simulink model "lab03fig2a"  (R2015a)
settings: Solver=ode45  StartTime=0.0  StopTime=20.0  RelTol=1e-3
settings Model: Creator=dg  LastModifiedBy=dg

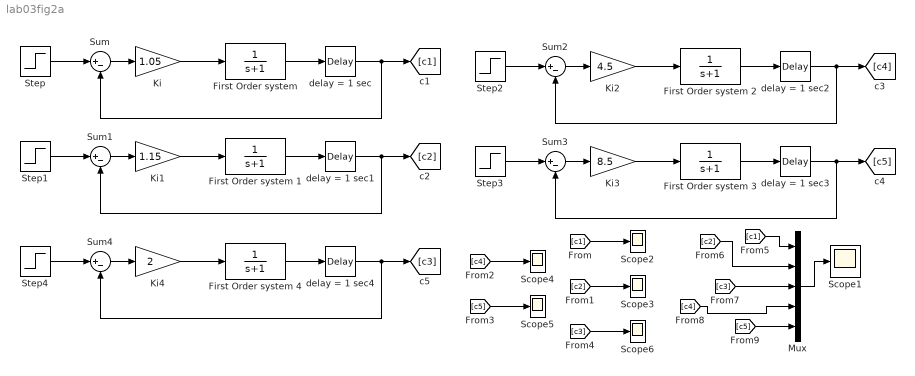
== system lab03fig2a ==
  First Order system {,1..4} (5 alike) : TransferFcn  Denominator=[1 1]
  Ki : Gain  Gain=1.05
  Ki1 : Gain  Gain=1.15
  Ki2 : Gain  Gain=4.5
  Ki3 : Gain  Gain=8.5
  Ki4 : Gain  Gain=2
  Mux : Mux  Inputs=5
  Scope{1..6} (6 alike) : Scope
      Scope1 settings: TickLabels=on  YMin=-1  YMax=4
      Scope2 settings: TickLabels=on  YMin=-1  YMax=4
      Scope3 settings: TickLabels=on  YMin=-1  YMax=4  SaveName=ScopeData2
      Scope4 settings: TickLabels=on  YMin=-1  YMax=4  SaveName=ScopeData3
      Scope5 settings: TickLabels=on  YMin=-1  YMax=4  SaveName=ScopeData4
      Scope6 settings: TickLabels=on  YMin=-1  YMax=4  SaveName=ScopeData5
  Step{,1..4} (5 alike) : Step  SampleTime=0
  Sum{,1..4} (5 alike) : Sum  Inputs=|+-
  delay = 1 sec{,1..4} (5 alike) : TransportDelay
  wires:
  Step/1 -> Sum/1
  Sum/1 -> Ki/1
  Ki/1 -> "First Order system "/1
  "First Order system "/1 -> delay = 1 sec/1
  delay = 1 sec/1 -> [c1], Sum/2
  Step1/1 -> Sum1/1
  Sum1/1 -> Ki1/1
  Ki1/1 -> First Order system 1/1
  First Order system 1/1 -> delay = 1 sec1/1
  delay = 1 sec1/1 -> [c2], Sum1/2
  Step2/1 -> Sum2/1
  Sum2/1 -> Ki2/1
  Ki2/1 -> First Order system 2/1
  First Order system 2/1 -> delay = 1 sec2/1
  delay = 1 sec2/1 -> [c4], Sum2/2
  Step3/1 -> Sum3/1
  Sum3/1 -> Ki3/1
  Ki3/1 -> First Order system 3/1
  First Order system 3/1 -> delay = 1 sec3/1
  delay = 1 sec3/1 -> [c5], Sum3/2
  Step4/1 -> Sum4/1
  Sum4/1 -> Ki4/1
  Ki4/1 -> First Order system 4/1
  First Order system 4/1 -> delay = 1 sec4/1
  delay = 1 sec4/1 -> [c3], Sum4/2
  [c1] -> Scope2/1
  Mux/1 -> Scope1/1
  [c2] -> Scope3/1
  [c3] -> Scope6/1
  [c4] -> Scope4/1
  [c5] -> Scope5/1
  [c1] -> Mux/1
  [c2] -> Mux/2
  [c3] -> Mux/3
  [c4] -> Mux/4
  [c5] -> Mux/5
